simulink model "Lift"  (R2020b)
settings: Solver=VariableStepAuto  StartTime=0.0  StopTime=100  RelTol=1e-3
settings Model: Creator=abhin  LastModifiedBy=abhin

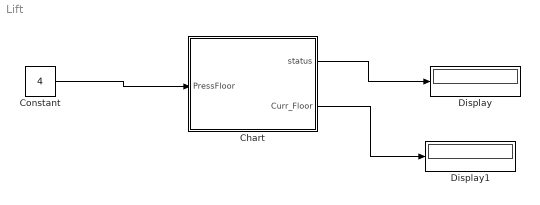
== system Lift ==
  Chart : Stateflow chart  TreatAsAtomicUnit=on
  Constant : Constant  Value=4
  Display : Display
  Display1 : Display
  wires:
  Constant/1 -> Chart/1(PressFloor)
  Chart/1(status) -> Display/1
  Chart/2(Curr_Floor) -> Display1/1

== stateflow chart Lift/Chart ==
  state LiftOperation
    entry:
    status=0;
    state LiftOn [parallel]
      entry:
      status=1;
      settings: executionOrder=1
      state GroundFloor
        entry:
        status=1;
        during:
        Curr_Floor=0;
        FloorCheck(Curr_Floor);
        exit:
        status=0;
      state FirstFloor
        entry:
        status=1;
        during:
        Curr_Floor=1;
        FloorCheck(Curr_Floor);
        exit:
        status=0;
      state SecondFloor
        entry:
        status=1;
        during:
        Curr_Floor=2;
        FloorCheck(Curr_Floor);
        exit:
        status=0;
      state ThirdFloor
        entry:
        status=1;
        during:
        Curr_Floor=3;
        FloorCheck(Curr_Floor);
        exit:
        status=0;
      state FourthFloor
        entry:
        status=1;
        during:
        Curr_Floor=4;
        FloorCheck(Curr_Floor);
        exit:
        status=0;
      state FifthFloor
        entry:
        status=1;
        during:
        Curr_Floor=5;
        FloorCheck(Curr_Floor);
        exit:
        status=0;
      (default) -> GroundFloor
      FirstFloor -> GroundFloor [order 1] : down
      GroundFloor -> FirstFloor : up
      SecondFloor -> FirstFloor [order 1] : down
      FirstFloor -> SecondFloor [order 2] : up
      ThirdFloor -> SecondFloor [order 1] : down
      SecondFloor -> ThirdFloor [order 2] : up
      FourthFloor -> ThirdFloor [order 1] : down
      ThirdFloor -> FourthFloor [order 2] : up
      FifthFloor -> FourthFloor : down
      FourthFloor -> FifthFloor [order 2] : up
    state LiftOff [parallel]
      entry:
      status=0;
      settings: executionOrder=2
  state FloorCheck(Floor) [function]
    (default) -> (junction 53)
    (junction 53) -> (junction 61) [order 3] : [PressFloor<Floor]
        | {send(down);
        | disp('GoingDown');}
    (junction 53) -> (junction 57) [order 1] : [PressFloor>Floor]
        | {send(up);
        | disp('GoingUp');}
    (junction 53) -> (junction 59) [order 2] : [PressFloor==Floor]
        | {disp('Current Floor');}
  (default) -> LiftOperation
  data: Floor function_input; status output; PressFloor input; Curr_Floor output
  events: down local RISING_EDGE_EVENT; up local RISING_EDGE_EVENT
